simulink model "smP5"  (R2023a)
settings: Solver=VariableStepAuto  StartTime=0.0  StopTime=0.005  RelTol=1e-3
model workspace (MAT data in the model file):
  C = 1e-07
  L = 0.006
  R = 100

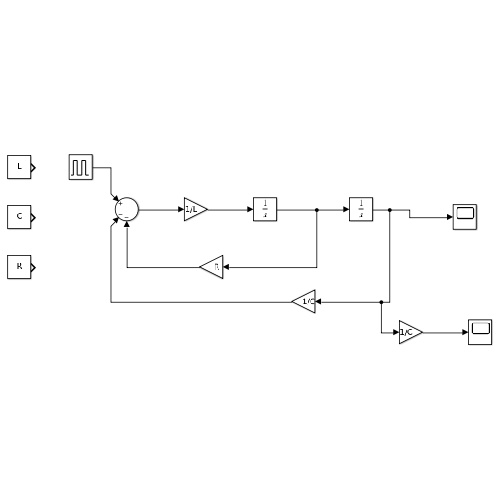
[thumbnail: Simulink's stored preview of the top-level diagram]
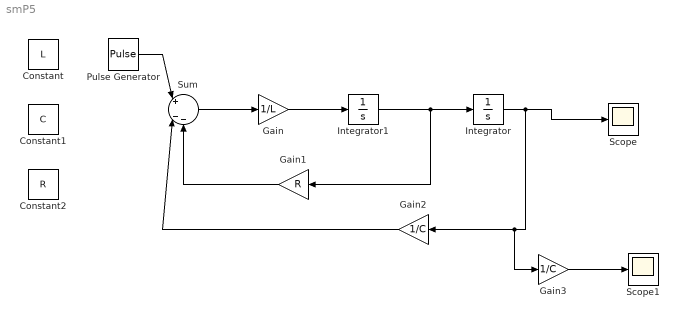
== system smP5 ==
  Constant : Constant  Value=L
  Constant1 : Constant  Value=C
  Constant2 : Constant  Value=R
  Gain : Gain  Gain=1/L
  Gain1 : Gain  Gain=R
  Gain2 : Gain  Gain=1/C
  Gain3 : Gain  Gain=1/C
  Integrator : Integrator
  Integrator1 : Integrator
  Pulse Generator : DiscretePulseGenerator  PulseType=Time based  Amplitude=5  Period=1/500  PulseWidth=50
  Scope : Scope
  Scope1 : Scope
  Sum : Sum  Inputs=|+|--
  wires:
  Sum/1 -> Gain/1
  Gain/1 -> Integrator1/1
  Integrator1/1 -> Gain1/1, Integrator/1
  Integrator/1 -> Gain3/1, Gain2/1, Scope/1
  Pulse Generator/1 -> Sum/1
  Gain1/1 -> Sum/3
  Gain2/1 -> Sum/2
  Gain3/1 -> Scope1/1
